simulink model "SVPWM_PMSM"  (Simulink 8.3)
settings: Solver=ode45  StartTime=0.0  StopTime=0.5  FixedStep=5e-6  RelTol=1e-3  AbsTol=1e-6
libraries: simulink x2
settings Model: Creator=ms09173  LastModifiedBy=wuyu
settings SolverCC: ConsecutiveZCsStepRelTol=100*128*eps  MaxConsecutiveZCs=1000000000
settings DataIOCC: SignalLoggingName=sigsOut
settings OptimizationCC: ExpressionDepthLimit=2147483647
settings DebuggingCC: SaveWithParameterizedLinksMsg=none  SignalResolutionControl=TryResolveAllWithWarning  SolverPrmCheckMsg=none  MultiTaskDSMMsg=warning  MultiTaskCondExecSysMsg=none  FcnCallInpInsideContextMsg=UseLocalSettings
settings HardwareCC: TargetUnknown=on
settings RTWCC: IncludeERTFirstTime=on

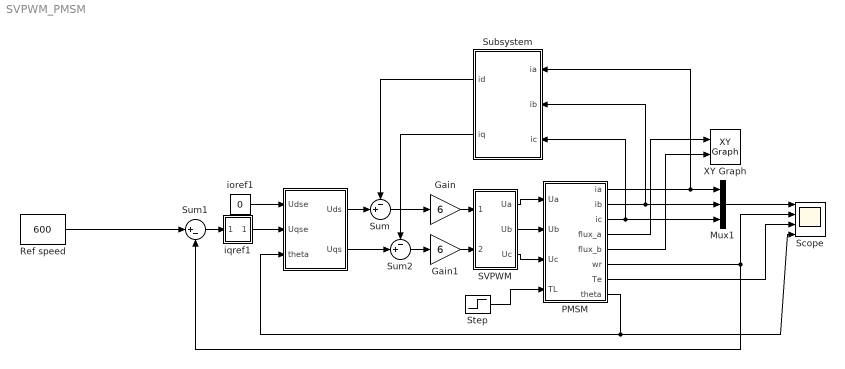
== system SVPWM_PMSM ==
  "                                      " : Subsystem
      mask Display:
      | disp('2r\n to\n  2s ');
      | port_label('output', 1, '\itI_a_s','texmode','on');
      | port_label('output', 2, '\itI_b_s','texmode','on');
      | port_label('input', 1, '\itI_{dse}','texmode','on');
      | port_label('input', 2, '\itI_{qse}','texmode','on');
      | port_label('input', 3, '\it\theta_m','texmode','on');
  Gain : Gain  Gain=6
  Gain1 : Gain  Gain=6
  Mux1 : Mux  Inputs=3
  PMSM : Subsystem  mask{Ld=8.5e-3, Lq=8.5e-3, r=2.875, flux_r=0.175, np=4, J=0.8e-3}
  Ref speed : Constant  Value=600
  SVPWM : Subsystem  mask{Ts=0.00005, Udc=310}
      mask prompts: Ts "Period of PWM(Ts):"; Udc "Voltage of DC(Udc):"
  Scope : Scope  NumInputPorts=4
      settings: TimeRange=0.3  YMin=-4~29.9874~4.97~1.7  YMax=4~29.9884~5.03~2.7  SaveName=v  MaxDataPoints=50000
  Step : Step  Time=0.15  Before=5  After=8  SampleTime=0
  Subsystem : Subsystem
      mask Display:
      | disp('3s\n to\n 2s ');
      | port_label('output', 1, '\iti_a_s','texmode','on');
      | port_label('output', 2, '\iti_b_s','texmode','on');
      | port_label('input', 1, '\iti_{as}','texmode','on');
      | port_label('input', 2, '\iti_{bs}','texmode','on');
      | port_label('input', 3, '\iti_{cs}','texmode','on');
  Sum : Sum  Inputs=-+|
  Sum1 : Sum  Inputs=|+-  SaturateOnIntegerOverflow=on
  Sum2 : Sum  Inputs=-+|
  XY Graph : simulink/Sinks/XY Graph  xmin=-0.3  xmax=0.3  ymin=-0.3  ymax=0.3  st=50e-6
  ioref1 : Constant  Value=0
  iqref1 : Subsystem  mask(PI Controller){I=40, P=500, sat=[-30, 30]}
      mask prompts: I "Integral"; P "Proportional:"; sat "Minimum and maximum outputs:"
      mask init:
      | min=sat(1);max=sat(2);
      mask Display: disp('PI')
  wires:
  Sum1/1 -> iqref1/1(In_1)
  iqref1/1(Out_1) -> "                                      "/2(Uqse)
  ioref1/1 -> "                                      "/1(Udse)
  SVPWM/1(Ua) -> PMSM/1(Ua)
  SVPWM/2(Ub) -> PMSM/2(Ub)
  SVPWM/3(Uc) -> PMSM/3(Uc)
  Step/1 -> PMSM/4(TL)
  PMSM/8(theta) -> "                                      "/3(theta), Scope/4
  PMSM/6(wr) -> Sum1/2, Scope/2
  PMSM/1(ia) -> Mux1/1, Subsystem/1(ia)
  PMSM/2(ib) -> Mux1/2, Subsystem/2(ib)
  PMSM/3(ic) -> Mux1/3, Subsystem/3(ic)
  Mux1/1 -> Scope/1
  PMSM/7(Te) -> Scope/3
  PMSM/4(flux_a) -> XY Graph/1
  PMSM/5(flux_b) -> XY Graph/2
  Subsystem/1(id) -> Sum/1
  "                                      "/1(Uds) -> Sum/2
  Subsystem/2("iq\t") -> Sum2/1
  "                                      "/2(Uqs) -> Sum2/2
  Sum/1 -> Gain/1
  Gain/1 -> SVPWM/1(Ualfa)
  Sum2/1 -> Gain1/1
  Gain1/1 -> SVPWM/2(Ubeta)
  Ref speed/1 -> Sum1/1

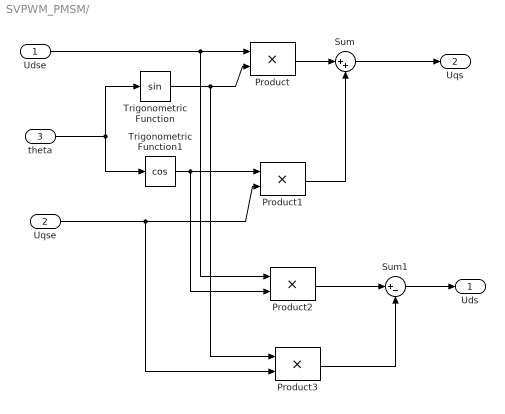
== system SVPWM_PMSM/                                       ==
  Udse : Inport
  Uqse : Inport  Port=2
  theta : Inport  Port=3
  Product{,1..3} (4 alike) : Product  SaturateOnIntegerOverflow=on  OutDataTypeStr=Inherit: Same as first input
  Sum : Sum  Inputs=|++  SaturateOnIntegerOverflow=on
  Sum1 : Sum  Inputs=|+-  SaturateOnIntegerOverflow=on
  Trigonometric Function : Trigonometry
  Trigonometric Function1 : Trigonometry  Operator=cos
  Uds : Outport
  Uqs : Outport  Port=2
  wires:
  Sum1/1 -> Uds/1
  Product3/1 -> Sum1/2
  Product2/1 -> Sum1/1
  Sum/1 -> Uqs/1
  Product1/1 -> Sum/2
  Product/1 -> Sum/1
  Uqse/1 -> Product1/2, Product3/2
  Trigonometric Function1/1 -> Product2/2, Product1/1
  Udse/1 -> Product/1, Product2/1
  Trigonometric Function/1 -> Product3/1, Product/2
  theta/1 -> Trigonometric Function/1, Trigonometric Function1/1

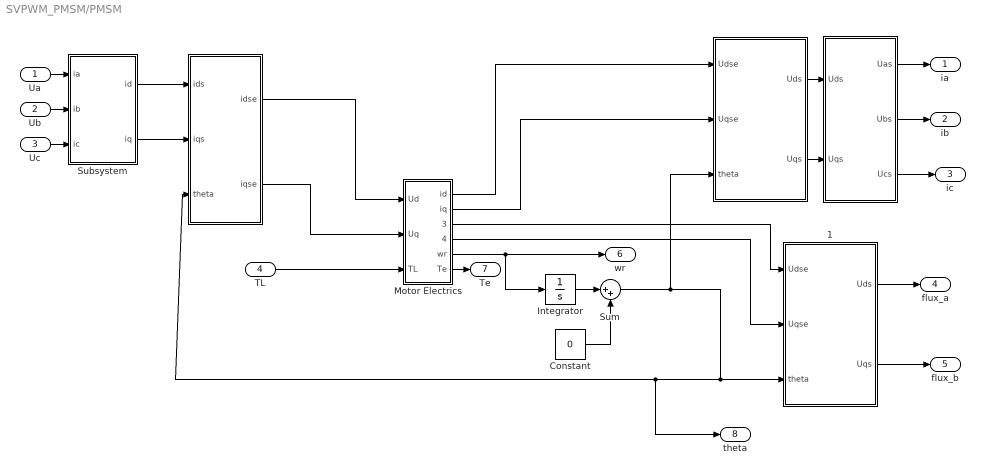
== system SVPWM_PMSM/PMSM ==
  Ua : Inport
  Ub : Inport  Port=2
  Uc : Inport  Port=3
  TL : Inport  Port=4
  "        " : Subsystem
      mask Display:
      | disp('2s\n to\n 2r ');
      | port_label('output', 1, '\iti_d_s_e','texmode','on');
      | port_label('output', 2, '\iti_q_s_e','texmode','on');
      | port_label('input', 1, '\iti_{ds}','texmode','on');
      | port_label('input', 2, '\iti_{qs}','texmode','on');
      | port_label('input', 3, '\it\theta_m','texmode','on');
  "                           " : Subsystem
      mask Display:
      | disp('2s\n to \n 3s ');
      | port_label('output', 1, '\itu_a','texmode','on');
      | port_label('output', 2, '\itu_b','texmode','on');
      | port_label('output', 3, '\itu_c','texmode','on');
      | port_label('input', 1, '\itV_{ds}','texmode','on');
      | port_label('input', 2, '\itV_{qs}','texmode','on');
  "                                      " : Subsystem
      mask Display:
      | disp('2r\n to\n  2s ');
      | port_label('output', 1, '\itu_d_s','texmode','on');
      | port_label('output', 2, '\itu_q_s','texmode','on');
      | port_label('input', 1, '\itV_{dse}','texmode','on');
      | port_label('input', 2, '\itV_{qse}','texmode','on');
      | port_label('input', 3, '\it\theta_m','texmode','on');
  "                                      1" : Subsystem
      mask Display:
      | disp('2r\n to\n  2s ');
      | port_label('output', 1, '\itu_d_s','texmode','on');
      | port_label('output', 2, '\itu_q_s','texmode','on');
      | port_label('input', 1, '\itV_{dse}','texmode','on');
      | port_label('input', 2, '\itV_{qse}','texmode','on');
      | port_label('input', 3, '\it\theta_m','texmode','on');
  Constant : Constant  Value=0
  Integrator : Integrator
  Motor Electrics : Subsystem
  Subsystem : Subsystem
      mask Display:
      | disp('3s\n to\n 2s ');
      | port_label('output', 1, '\iti_d_s','texmode','on');
      | port_label('output', 2, '\iti_q_s','texmode','on');
      | port_label('input', 1, '\iti_{as}','texmode','on');
      | port_label('input', 2, '\iti_{bs}','texmode','on');
      | port_label('input', 3, '\iti_{cs}','texmode','on');
  Sum : Sum  Inputs=|++  SaturateOnIntegerOverflow=on
  ia : Outport
  ib : Outport  Port=2
  ic : Outport  Port=3
  flux_a : Outport  Port=4
  flux_b : Outport  Port=5
  wr : Outport  Port=6
  Te : Outport  Port=7
  theta : Outport  Port=8
  wires:
  Motor Electrics/6(Te) -> Te/1
  Motor Electrics/4(flux_q) -> "                                      1"/2(Uqse)
  "                                      1"/2(Uqs) -> flux_b/1
  "                                      1"/1(Uds) -> flux_a/1
  "                           "/3(Ucs) -> ic/1
  "                           "/2(Ubs) -> ib/1
  "                           "/1(Uas) -> ia/1
  "                                      "/2(Uqs) -> "                           "/2(Uqs)
  "                                      "/1(Uds) -> "                           "/1(Uds)
  Motor Electrics/2(iq) -> "                                      "/2(Uqse)
  Motor Electrics/1(id) -> "                                      "/1(Udse)
  Sum/1 -> theta/1, "        "/3(theta), "                                      1"/3(theta), "                                      "/3(theta)
  Constant/1 -> Sum/2
  Integrator/1 -> Sum/1
  Uc/1 -> Subsystem/3(ic)
  Ub/1 -> Subsystem/2(ib)
  Ua/1 -> Subsystem/1(ia)
  "        "/2(iqse) -> Motor Electrics/2(Uq)
  "        "/1(idse) -> Motor Electrics/1(Ud)
  Subsystem/2("iq\t") -> "        "/2(iqs)
  Subsystem/1(id) -> "        "/1(ids)
  TL/1 -> Motor Electrics/3(TL)
  Motor Electrics/5(wr) -> wr/1, Integrator/1
  Motor Electrics/3(flux_d) -> "                                      1"/1(Udse)

== system SVPWM_PMSM/SVPWM ==
  Ualfa : Inport
  Ubeta : Inport  Port=2
  Constant : Constant  Value=Udc
  Constant1 : Constant  Value=Ts
  N1 : Subsystem
  Subsystem : Subsystem
  Subsystem1 : Subsystem
  X.Y.Z : Subsystem
  produce PWM : Subsystem
  Ua : Outport
  Ub : Outport  Port=2
  Uc : Outport  Port=3
  wires:
  Constant1/1 -> X.Y.Z/1(T), Subsystem1/3(T), Subsystem/5(T)
  Constant/1 -> X.Y.Z/4(Udc)
  N1/1(N) -> Subsystem1/4(N), Subsystem/1(N)
  X.Y.Z/1(X) -> Subsystem/2(X)
  X.Y.Z/2(Y) -> Subsystem/3(Y)
  X.Y.Z/3(Z) -> Subsystem/4(Z)
  Subsystem1/1(Tcm1) -> produce PWM/1(Tcm1)
  Subsystem1/2(Tcm2) -> produce PWM/2(Tcm2)
  Subsystem1/3(Tcm3) -> produce PWM/3(Tcm3)
  Ualfa/1 -> X.Y.Z/2(Ualfa), N1/1(Ualfa)
  Subsystem/1(T1) -> Subsystem1/1(T1)
  Subsystem/2(T2) -> Subsystem1/2(T2)
  Ubeta/1 -> N1/2(Ubeta), X.Y.Z/3(Ubeta)
  produce PWM/2(Ub) -> Ub/1
  produce PWM/1(Ua) -> Ua/1
  produce PWM/3(Uc) -> Uc/1

== system SVPWM_PMSM/Subsystem ==
  ia : Inport
  ib : Inport  Port=2
  ic : Inport  Port=3
  Gain : Gain  Gain=-1/2  SaturateOnIntegerOverflow=on  OutDataTypeStr=Inherit: Same as input  ParamDataTypeStr=Inherit: Same as input
  Gain1 : Gain  Gain=sqrt(2/3)  SaturateOnIntegerOverflow=on  OutDataTypeStr=Inherit: Same as input  ParamDataTypeStr=Inherit: Same as input
  Gain2 : Gain  Gain=sqrt(2)/2  SaturateOnIntegerOverflow=on  OutDataTypeStr=Inherit: Same as input  ParamDataTypeStr=Inherit: Same as input
  Sum : Sum  Inputs=|++  SaturateOnIntegerOverflow=on
  Sum1 : Sum  Inputs=|++  SaturateOnIntegerOverflow=on
  Sum2 : Sum  Inputs=|-+  SaturateOnIntegerOverflow=on
  id : Outport
  "iq\t" : Outport  Port=2
  wires:
  Gain2/1 -> "iq\t"/1
  Sum2/1 -> Gain2/1
  ib/1 -> Sum/1, Sum2/2
  ic/1 -> Sum2/1, Sum/2
  Gain1/1 -> id/1
  Sum1/1 -> Gain1/1
  Gain/1 -> Sum1/2
  ia/1 -> Sum1/1
  Sum/1 -> Gain/1

== system SVPWM_PMSM/iqref1 ==
  In_1 : Inport  PortDimensions=1
  Integral : TransferFcn  Numerator=[I]  Denominator=[1 0]
  Proportional : Gain  Gain=P  SaturateOnIntegerOverflow=on  OutDataTypeStr=Inherit: Same as input  ParamDataTypeStr=Inherit: Same as input
  Saturation : Saturate  UpperLimit=max  LowerLimit=min
  Sum : Sum  SaturateOnIntegerOverflow=on  InputSameDT=on  OutDataTypeStr=Inherit: Same as first input
  Out_1 : Outport  InitialOutput=0
  wires:
  Integral/1 -> Sum/2
  In_1/1 -> Integral/1, Proportional/1
  Proportional/1 -> Sum/1
  Sum/1 -> Saturation/1
  Saturation/1 -> Out_1/1

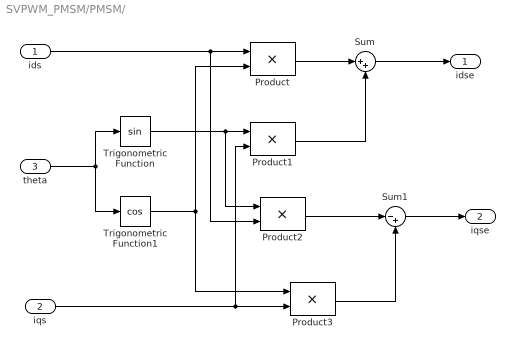
== system SVPWM_PMSM/PMSM/         ==
  ids : Inport
  iqs : Inport  Port=2
  theta : Inport  Port=3
  Product{,1..3} (4 alike) : Product  SaturateOnIntegerOverflow=on  OutDataTypeStr=Inherit: Same as first input
  Sum : Sum  Inputs=|++  SaturateOnIntegerOverflow=on
  Sum1 : Sum  Inputs=|-+  SaturateOnIntegerOverflow=on
  Trigonometric Function : Trigonometry
  Trigonometric Function1 : Trigonometry  Operator=cos
  idse : Outport
  iqse : Outport  Port=2
  wires:
  Sum1/1 -> iqse/1
  Product3/1 -> Sum1/2
  Product2/1 -> Sum1/1
  Sum/1 -> idse/1
  Product1/1 -> Sum/2
  Product/1 -> Sum/1
  iqs/1 -> Product1/2, Product3/2
  Trigonometric Function/1 -> Product2/1, Product1/1
  Trigonometric Function1/1 -> Product3/1, Product/2
  ids/1 -> Product/1, Product2/2
  theta/1 -> Trigonometric Function/1, Trigonometric Function1/1

== system SVPWM_PMSM/PMSM/                            ==
  Uds : Inport
  Uqs : Inport  Port=2
  Gain : Gain  Gain=sqrt(2/3)  SaturateOnIntegerOverflow=on  OutDataTypeStr=Inherit: Same as input  ParamDataTypeStr=Inherit: Same as input
  Gain1 : Gain  Gain=1/2  SaturateOnIntegerOverflow=on  OutDataTypeStr=Inherit: Same as input  ParamDataTypeStr=Inherit: Same as input
  Gain2 : Gain  Gain=sqrt(3)/2  SaturateOnIntegerOverflow=on  OutDataTypeStr=Inherit: Same as input  ParamDataTypeStr=Inherit: Same as input
  Gain3 : Gain  Gain=sqrt(2/3)  SaturateOnIntegerOverflow=on  OutDataTypeStr=Inherit: Same as input  ParamDataTypeStr=Inherit: Same as input
  Gain4 : Gain  Gain=sqrt(2/3)  SaturateOnIntegerOverflow=on  OutDataTypeStr=Inherit: Same as input  ParamDataTypeStr=Inherit: Same as input
  Sum : Sum  Inputs=|-+  SaturateOnIntegerOverflow=on
  Sum1 : Sum  Inputs=|--  SaturateOnIntegerOverflow=on
  Uas : Outport
  Ubs : Outport  Port=2
  Ucs : Outport  Port=3
  wires:
  Gain4/1 -> Ucs/1
  Sum1/1 -> Gain4/1
  Gain3/1 -> Ubs/1
  Sum/1 -> Gain3/1
  Gain2/1 -> Sum1/1, Sum/2
  Gain1/1 -> Sum1/2, Sum/1
  Uqs/1 -> Gain2/1
  Uds/1 -> Gain/1, Gain1/1
  Gain/1 -> Uas/1

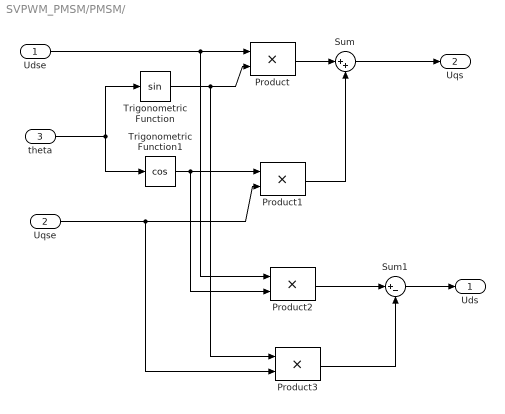
== system SVPWM_PMSM/PMSM/                                       ==
  Udse : Inport
  Uqse : Inport  Port=2
  theta : Inport  Port=3
  Product{,1..3} (4 alike) : Product  SaturateOnIntegerOverflow=on  OutDataTypeStr=Inherit: Same as first input
  Sum : Sum  Inputs=|++  SaturateOnIntegerOverflow=on
  Sum1 : Sum  Inputs=|+-  SaturateOnIntegerOverflow=on
  Trigonometric Function : Trigonometry
  Trigonometric Function1 : Trigonometry  Operator=cos
  Uds : Outport
  Uqs : Outport  Port=2
  wires:
  Sum1/1 -> Uds/1
  Product3/1 -> Sum1/2
  Product2/1 -> Sum1/1
  Sum/1 -> Uqs/1
  Product1/1 -> Sum/2
  Product/1 -> Sum/1
  Uqse/1 -> Product1/2, Product3/2
  Trigonometric Function1/1 -> Product2/2, Product1/1
  Udse/1 -> Product/1, Product2/1
  Trigonometric Function/1 -> Product3/1, Product/2
  theta/1 -> Trigonometric Function/1, Trigonometric Function1/1

== system SVPWM_PMSM/PMSM/                                      1 ==
  Udse : Inport
  Uqse : Inport  Port=2
  theta : Inport  Port=3
  Product{,1..3} (4 alike) : Product  SaturateOnIntegerOverflow=on  OutDataTypeStr=Inherit: Same as first input
  Sum : Sum  Inputs=|++  SaturateOnIntegerOverflow=on
  Sum1 : Sum  Inputs=|+-  SaturateOnIntegerOverflow=on
  Trigonometric Function : Trigonometry
  Trigonometric Function1 : Trigonometry  Operator=cos
  Uds : Outport
  Uqs : Outport  Port=2
  wires:
  theta/1 -> Trigonometric Function1/1, Trigonometric Function/1
  Trigonometric Function/1 -> Product/2, Product3/1
  Udse/1 -> Product2/1, Product/1
  Trigonometric Function1/1 -> Product1/1, Product2/2
  Uqse/1 -> Product3/2, Product1/2
  Product/1 -> Sum/1
  Product1/1 -> Sum/2
  Sum/1 -> Uqs/1
  Product2/1 -> Sum1/1
  Product3/1 -> Sum1/2
  Sum1/1 -> Uds/1

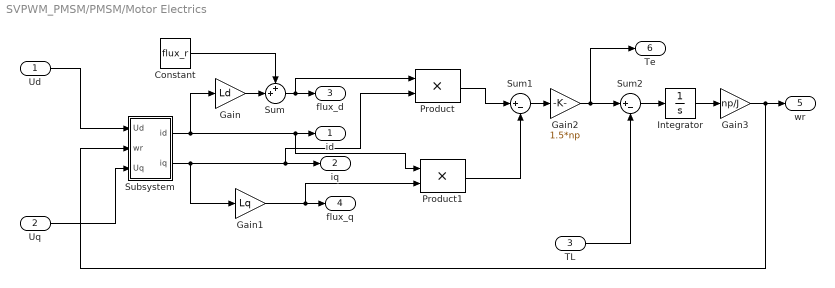
== system SVPWM_PMSM/PMSM/Motor Electrics ==
  Ud : Inport
  Uq : Inport  Port=2
  TL : Inport  Port=3
  Constant : Constant  Value=flux_r
  Gain : Gain  Gain=Ld  SaturateOnIntegerOverflow=on  OutDataTypeStr=Inherit: Same as input  ParamDataTypeStr=Inherit: Same as input
  Gain1 : Gain  Gain=Lq  SaturateOnIntegerOverflow=on  OutDataTypeStr=Inherit: Same as input  ParamDataTypeStr=Inherit: Same as input
  Gain2 : Gain  Gain=1.5*np  SaturateOnIntegerOverflow=on  OutDataTypeStr=Inherit: Same as input  ParamDataTypeStr=Inherit: Same as input
  Gain3 : Gain  Gain=np/J  SaturateOnIntegerOverflow=on  OutDataTypeStr=Inherit: Same as input  ParamDataTypeStr=Inherit: Same as input
  Integrator : Integrator
  Product : Product  SaturateOnIntegerOverflow=on  OutDataTypeStr=Inherit: Same as first input
  Product1 : Product  SaturateOnIntegerOverflow=on  OutDataTypeStr=Inherit: Same as first input
  Subsystem : Subsystem
  Sum : Sum  Inputs=++|  SaturateOnIntegerOverflow=on
  Sum1 : Sum  Inputs=|+-  SaturateOnIntegerOverflow=on
  Sum2 : Sum  Inputs=|+-  SaturateOnIntegerOverflow=on
  id : Outport
  iq : Outport  Port=2
  flux_d : Outport  Port=3
  flux_q : Outport  Port=4
  wr : Outport  Port=5
  Te : Outport  Port=6
  wires:
  Gain3/1 -> wr/1, Subsystem/2(wr)
  Integrator/1 -> Gain3/1
  Sum2/1 -> Integrator/1
  TL/1 -> Sum2/2
  Gain2/1 -> Te/1, Sum2/1
  Sum1/1 -> Gain2/1
  Product1/1 -> Sum1/2
  Product/1 -> Sum1/1
  Gain1/1 -> Product1/2, flux_q/1
  Sum/1 -> Product/1, flux_d/1
  Constant/1 -> Sum/1
  Gain/1 -> Sum/2
  Uq/1 -> Subsystem/3(Uq)
  Subsystem/2(iq) -> Product/2, iq/1, Gain1/1
  Ud/1 -> Subsystem/1(Ud)
  Subsystem/1(id) -> Product1/1, id/1, Gain/1

== system SVPWM_PMSM/PMSM/Subsystem ==
  ia : Inport
  ib : Inport  Port=2
  ic : Inport  Port=3
  Gain : Gain  Gain=-1/2  SaturateOnIntegerOverflow=on  OutDataTypeStr=Inherit: Same as input  ParamDataTypeStr=Inherit: Same as input
  Gain1 : Gain  Gain=sqrt(2/3)  SaturateOnIntegerOverflow=on  OutDataTypeStr=Inherit: Same as input  ParamDataTypeStr=Inherit: Same as input
  Gain2 : Gain  Gain=sqrt(2)/2  SaturateOnIntegerOverflow=on  OutDataTypeStr=Inherit: Same as input  ParamDataTypeStr=Inherit: Same as input
  Sum : Sum  Inputs=|++  SaturateOnIntegerOverflow=on
  Sum1 : Sum  Inputs=|++  SaturateOnIntegerOverflow=on
  Sum2 : Sum  Inputs=|-+  SaturateOnIntegerOverflow=on
  id : Outport
  "iq\t" : Outport  Port=2
  wires:
  Gain2/1 -> "iq\t"/1
  Sum2/1 -> Gain2/1
  ib/1 -> Sum/1, Sum2/2
  ic/1 -> Sum2/1, Sum/2
  Gain1/1 -> id/1
  Sum1/1 -> Gain1/1
  Gain/1 -> Sum1/2
  ia/1 -> Sum1/1
  Sum/1 -> Gain/1

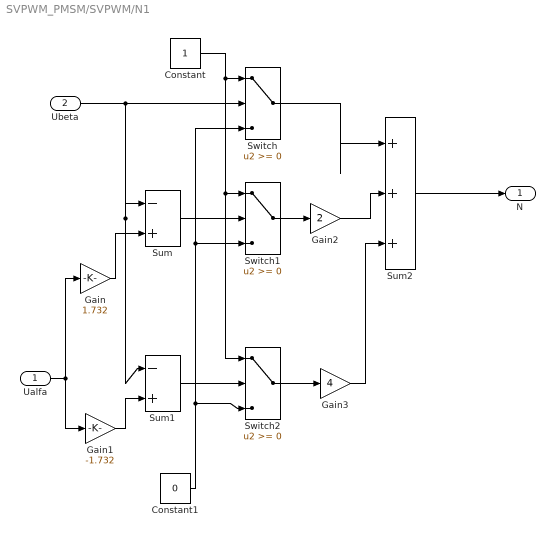
== system SVPWM_PMSM/SVPWM/N1 ==
  Ualfa : Inport
  Ubeta : Inport  Port=2
  Constant : Constant
  Constant1 : Constant  Value=0
  Gain : Gain  Gain=1.732
  Gain1 : Gain  Gain=-1.732
  Gain2 : Gain  Gain=2
  Gain3 : Gain  Gain=4
  Sum : Sum  Inputs=|-+
  Sum1 : Sum  Inputs=|-+
  Sum2 : Sum  Inputs=|+++
  Switch : Switch  ZeroCross=off
  Switch1 : Switch  ZeroCross=off
  Switch2 : Switch  ZeroCross=off
  N : Outport
  wires:
  Ubeta/1 -> Switch/2, Sum/1, Sum1/1
  Constant/1 -> Switch/1, Switch2/1, Switch1/1
  Ualfa/1 -> Gain1/1, Gain/1
  Gain/1 -> Sum/2
  Sum/1 -> Switch1/2
  Sum1/1 -> Switch2/2
  Gain1/1 -> Sum1/2
  Constant1/1 -> Switch/3, Switch1/3, Switch2/3
  Switch1/1 -> Gain2/1
  Switch2/1 -> Gain3/1
  Gain2/1 -> Sum2/2
  Switch/1 -> Sum2/1
  Gain3/1 -> Sum2/3
  Sum2/1 -> N/1

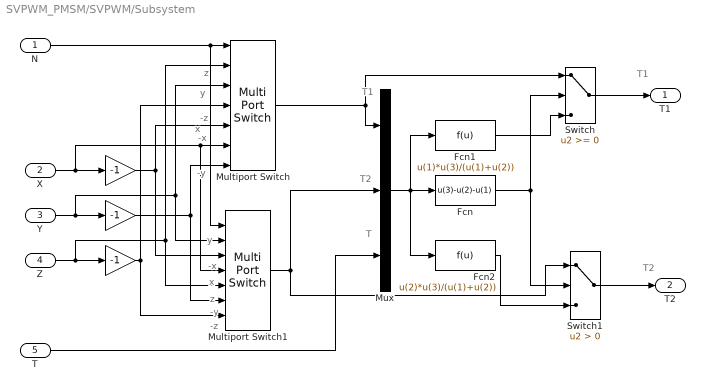
== system SVPWM_PMSM/SVPWM/Subsystem ==
  note: z
  note: y
  note: -z
  note: -x
  note: x
  note: -y
  note: y
  note: -x
  note: x
  note: z
  note: -y
  note: -z
  note: T1
  note: T2
  note: T
  note: T1
  note: T2
  N : Inport
  X : Inport  Port=2
  Y : Inport  Port=3
  Z : Inport  Port=4
  T : Inport  Port=5
  " " : Gain  Gain=-1
  "  " : Gain  Gain=-1
  "    " : Gain  Gain=-1
  Fcn : Fcn  Expr=u(3)-u(2)-u(1)
  Fcn1 : Fcn  Expr=u(1)*u(3)/(u(1)+u(2))
  Fcn2 : Fcn  Expr=u(2)*u(3)/(u(1)+u(2))
  Multiport Switch : MultiPortSwitch  Inputs=6
  Multiport Switch1 : MultiPortSwitch  Inputs=6
  Mux : Mux  Inputs=3
  Switch : Switch
  Switch1 : Switch  Criteria=u2 > Threshold
  T1 : Outport
  T2 : Outport  Port=2
  wires:
  N/1 -> Multiport Switch1/1, Multiport Switch/1
  X/1 -> Multiport Switch1/4, Multiport Switch/6, " "/1
  Y/1 -> Multiport Switch1/2, Multiport Switch/3, "  "/1
  Z/1 -> Multiport Switch1/5, Multiport Switch/2, "    "/1
  "    "/1 -> Multiport Switch1/7, Multiport Switch/4
  "  "/1 -> Multiport Switch/7, Multiport Switch1/6
  " "/1 -> Multiport Switch/5, Multiport Switch1/3
  Multiport Switch/1 -> Mux/1, Switch/1
  Multiport Switch1/1 -> Switch1/1, Mux/2
  T/1 -> Mux/3
  Mux/1 -> Fcn/1, Fcn1/1, Fcn2/1
  Fcn/1 -> Switch/2, Switch1/2
  Fcn1/1 -> Switch/3
  Fcn2/1 -> Switch1/3
  Switch/1 -> T1/1
  Switch1/1 -> T2/1

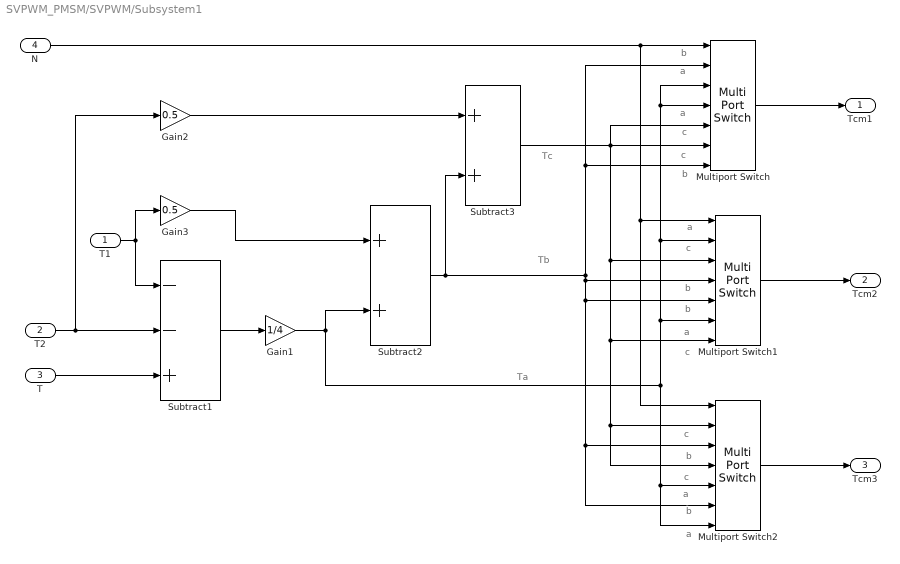
== system SVPWM_PMSM/SVPWM/Subsystem1 ==
  note: Ta
  note: Tb
  note: Tc
  note: b
  note: a
  note: a
  note: c
  note: c
  note: b
  note: a
  note: c
  note: b
  note: b
  note: a
  note: c
  note: c
  note: b
  note: c
  note: a
  note: b
  note: a
  T1 : Inport
  T2 : Inport  Port=2
  T : Inport  Port=3
  N : Inport  Port=4
  Gain1 : Gain  Gain=1/4
  Gain2 : Gain  Gain=0.5
  Gain3 : Gain  Gain=0.5
  Multiport Switch : MultiPortSwitch  Inputs=6
  Multiport Switch1 : MultiPortSwitch  Inputs=6
  Multiport Switch2 : MultiPortSwitch  Inputs=6
  Subtract1 : Sum  Inputs=--+
  Subtract2 : Sum
  Subtract3 : Sum
  Tcm1 : Outport
  Tcm2 : Outport  Port=2
  Tcm3 : Outport  Port=3
  wires:
  T2/1 -> Gain2/1, Subtract1/2
  T/1 -> Subtract1/3
  T1/1 -> Gain3/1, Subtract1/1
  Gain3/1 -> Subtract2/1
  Subtract1/1 -> Gain1/1
  Gain1/1 -> Subtract2/2, Multiport Switch/3, Multiport Switch/4, Multiport Switch1/2, Multiport Switch1/6, Multiport Switch2/5, Multiport Switch2/7
  Subtract2/1 -> Subtract3/2, Multiport Switch/2, Multiport Switch/7, Multiport Switch1/4, Multiport Switch1/5, Multiport Switch2/3, Multiport Switch2/6
  Gain2/1 -> Subtract3/1
  N/1 -> Multiport Switch/1, Multiport Switch2/1, Multiport Switch1/1
  Multiport Switch/1 -> Tcm1/1
  Multiport Switch1/1 -> Tcm2/1
  Multiport Switch2/1 -> Tcm3/1
  Subtract3/1 -> Multiport Switch/5, Multiport Switch/6, Multiport Switch1/3, Multiport Switch1/7, Multiport Switch2/2, Multiport Switch2/4

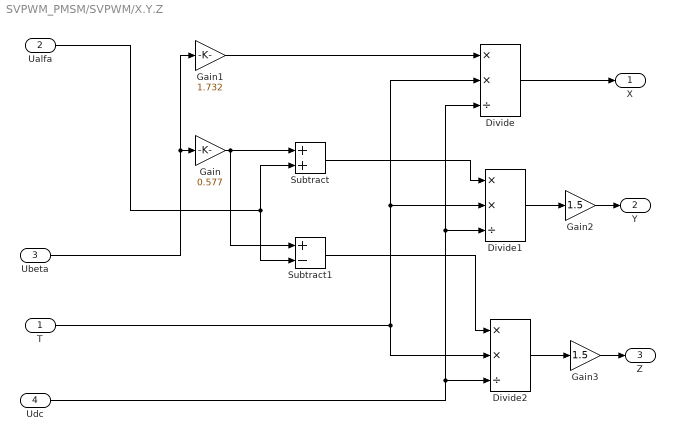
== system SVPWM_PMSM/SVPWM/X.Y.Z ==
  T : Inport
  Ualfa : Inport  Port=2
  Ubeta : Inport  Port=3
  Udc : Inport  Port=4
  Divide : Product  Inputs=**/
  Divide1 : Product  Inputs=**/
  Divide2 : Product  Inputs=**/
  Gain : Gain  Gain=0.577
  Gain1 : Gain  Gain=1.732
  Gain2 : Gain  Gain=1.5
  Gain3 : Gain  Gain=1.5
  Subtract : Sum
  Subtract1 : Sum  Inputs=+-
  X : Outport
  Y : Outport  Port=2
  Z : Outport  Port=3
  wires:
  Gain/1 -> Subtract/1, Subtract1/1
  Gain1/1 -> Divide/1
  T/1 -> Divide2/2, Divide1/2, Divide/2
  Udc/1 -> Divide2/3, Divide1/3, Divide/3
  Ualfa/1 -> Subtract1/2, Subtract/2
  Subtract/1 -> Divide1/1
  Subtract1/1 -> Divide2/1
  Divide/1 -> X/1
  Divide1/1 -> Gain2/1
  Divide2/1 -> Gain3/1
  Gain2/1 -> Y/1
  Gain3/1 -> Z/1
  Ubeta/1 -> Gain1/1, Gain/1

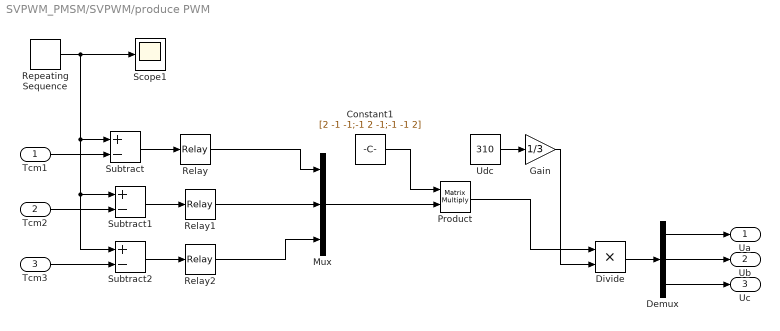
== system SVPWM_PMSM/SVPWM/produce PWM ==
  Tcm1 : Inport
  Tcm2 : Inport  Port=2
  Tcm3 : Inport  Port=3
  Constant1 : Constant  Value=[2 -1 -1;-1 2 -1;-1 -1 2]
  Demux : Demux  Outputs=3
  Divide : Product  Inputs=**
  Gain : Gain  Gain=1/3
  Mux : Mux  Inputs=3
  Product : Product  Multiplication=Matrix(*)  RndMeth=Zero
  Relay : Relay  OnSwitchValue=2e-10  OffSwitchValue=-2e-10
  Relay1 : Relay  OnSwitchValue=2e-10  OffSwitchValue=-2e-10
  Relay2 : Relay  OnSwitchValue=2e-10  OffSwitchValue=-2e-10
  Repeating Sequence : simulink/Sources/Repeating Sequence  rep_seq_t=[0 Ts/2 Ts]  rep_seq_y=[0 Ts/2 0]
  Scope1 : Scope
      settings: TimeRange=0.3  YMin=0  YMax=2.5e-005  SaveName=ScopeData6
  Subtract : Sum  Inputs=+-
  Subtract1 : Sum  Inputs=+-
  Subtract2 : Sum  Inputs=+-
  Udc : Constant  Value=310
  Ua : Outport
  Ub : Outport  Port=2
  Uc : Outport  Port=3
  wires:
  Subtract/1 -> Relay/1
  Subtract1/1 -> Relay1/1
  Subtract2/1 -> Relay2/1
  Repeating Sequence/1 -> Subtract/1, Subtract2/1, Subtract1/1, Scope1/1
  Tcm1/1 -> Subtract/2
  Tcm2/1 -> Subtract1/2
  Tcm3/1 -> Subtract2/2
  Udc/1 -> Gain/1
  Relay/1 -> Mux/1
  Relay1/1 -> Mux/2
  Relay2/1 -> Mux/3
  Constant1/1 -> Product/1
  Mux/1 -> Product/2
  Product/1 -> Divide/1
  Gain/1 -> Divide/2
  Divide/1 -> Demux/1
  Demux/1 -> Ua/1
  Demux/2 -> Ub/1
  Demux/3 -> Uc/1

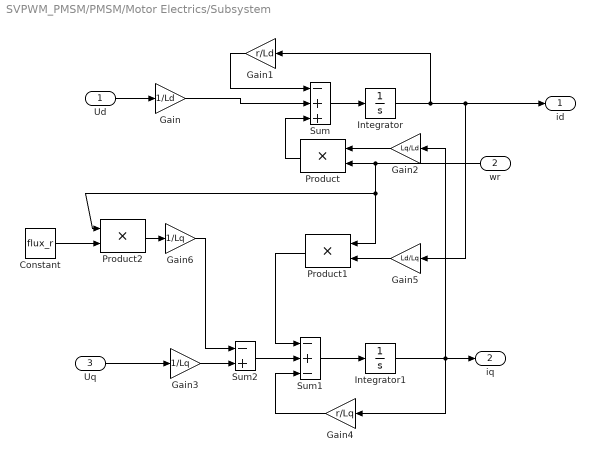
== system SVPWM_PMSM/PMSM/Motor Electrics/Subsystem ==
  Ud : Inport
  wr : Inport  Port=2
  Uq : Inport  Port=3
  Constant : Constant  Value=flux_r
  Gain : Gain  Gain=1/Ld  SaturateOnIntegerOverflow=on  OutDataTypeStr=Inherit: Same as input  ParamDataTypeStr=Inherit: Same as input
  Gain1 : Gain  Gain=r/Ld  SaturateOnIntegerOverflow=on  OutDataTypeStr=Inherit: Same as input  ParamDataTypeStr=Inherit: Same as input
  Gain2 : Gain  Gain=Lq/Ld  SaturateOnIntegerOverflow=on  OutDataTypeStr=Inherit: Same as input  ParamDataTypeStr=Inherit: Same as input
  Gain3 : Gain  Gain=1/Lq  SaturateOnIntegerOverflow=on  OutDataTypeStr=Inherit: Same as input  ParamDataTypeStr=Inherit: Same as input
  Gain4 : Gain  Gain=r/Lq  SaturateOnIntegerOverflow=on  OutDataTypeStr=Inherit: Same as input  ParamDataTypeStr=Inherit: Same as input
  Gain5 : Gain  Gain=Ld/Lq  SaturateOnIntegerOverflow=on  OutDataTypeStr=Inherit: Same as input  ParamDataTypeStr=Inherit: Same as input
  Gain6 : Gain  Gain=1/Lq  SaturateOnIntegerOverflow=on  OutDataTypeStr=Inherit: Same as input  ParamDataTypeStr=Inherit: Same as input
  Integrator : Integrator
  Integrator1 : Integrator
  Product : Product  SaturateOnIntegerOverflow=on  OutDataTypeStr=Inherit: Same as first input
  Product1 : Product  SaturateOnIntegerOverflow=on  OutDataTypeStr=Inherit: Same as first input
  Product2 : Product  SaturateOnIntegerOverflow=on  OutDataTypeStr=Inherit: Same as first input
  Sum : Sum  Inputs=-++  SaturateOnIntegerOverflow=on
  Sum1 : Sum  Inputs=-+-  SaturateOnIntegerOverflow=on
  Sum2 : Sum  Inputs=-+  SaturateOnIntegerOverflow=on
  id : Outport
  iq : Outport  Port=2
  wires:
  Gain6/1 -> Sum2/1
  Product2/1 -> Gain6/1
  Sum2/1 -> Sum1/2
  Gain3/1 -> Sum2/2
  Constant/1 -> Product2/2
  Integrator1/1 -> Gain4/1, Gain2/1, iq/1
  Product1/1 -> Sum1/1
  Gain5/1 -> Product1/2
  Gain4/1 -> Sum1/3
  wr/1 -> Product/2, Product1/1, Product2/1
  Product/1 -> Sum/3
  Gain2/1 -> Product/1
  Sum1/1 -> Integrator1/1
  Uq/1 -> Gain3/1
  Gain/1 -> Sum/2
  Gain1/1 -> Sum/1
  Sum/1 -> Integrator/1
  Integrator/1 -> Gain5/1, id/1, Gain1/1
  Ud/1 -> Gain/1
